simulink model "Aircraft6DSimulation"  (R2022a)
settings: Solver=FixedStepAuto  StartTime=0.0  StopTime=TF  FixedStep=dt  RelTol=1e-3
values from neighbouring files (symbols this model uses):
  a = 0    [run_model.m]
  e = 5*pi/180    (= 0.0872664625997)    [run_model.m]
  r = X(6)    [Dot_Model.m]    (also in run_model.m = out.simX.Data(:,6) * 180/pi)
  t1 = 10    [run_model.m]
  t2 = t1+2    (= 12)    [run_model.m]
  u0 = [-0.23791*pi/180 ... (first row only)    [run_model.m]
  x0 = [75 ... (first row only)    [run_model.m]
undefined symbols (not defined in the file or in its folder): Dot_Model
settings Model: Creator=Lemon  LastModifiedBy=Lemon
settings SolverCC: ZeroCrossControl=EnableAll  EnableFixedStepZeroCrossing=on

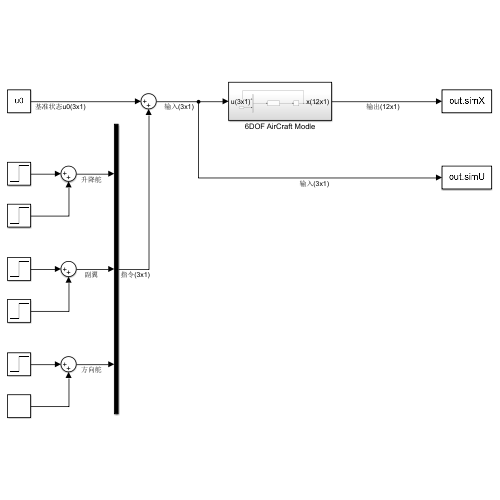
[thumbnail: Simulink's stored preview of the top-level diagram]
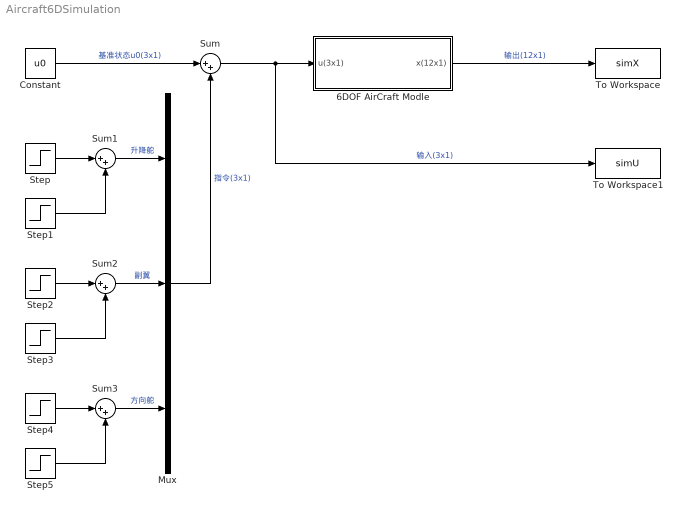
== system Aircraft6DSimulation ==
  6DOF AirCraft Modle : Subsystem
  Constant : Constant  Value=u0
  Mux : Mux  Inputs=3
  Step : Step  Time=t1  After=-e  SampleTime=0
  Step1 : Step  Time=t2  After=e  SampleTime=0
  Step2 : Step  Time=t1  After=a  SampleTime=0
  Step3 : Step  Time=t2  After=-a  SampleTime=0
  Step4 : Step  Time=t1  After=r  SampleTime=0
  Step5 : Step  Time=t2  After=-r  SampleTime=0
  Sum{,1..3} (4 alike) : Sum  Inputs=|++
  To Workspace : ToWorkspace  VariableName=simX  SaveFormat=Timeseries  SampleTime=-1
  To Workspace1 : ToWorkspace  VariableName=simU  SaveFormat=Timeseries  SampleTime=-1
  wires:
  6DOF AirCraft Modle/1(x(12x1)) -> To Workspace/1  "输出(12x1)"
  Constant/1 -> Sum/1  "基准状态u0(3x1)"
  Sum/1 -> To Workspace1/1, 6DOF AirCraft Modle/1(u(3x1))  "输入(3x1)"
  Mux/1 -> Sum/2  "指令(3x1)"
  Sum1/1 -> Mux/1  "升降舵"
  Step/1 -> Sum1/1
  Step1/1 -> Sum1/2
  Step2/1 -> Sum2/1
  Sum2/1 -> Mux/2  "副翼"
  Step3/1 -> Sum2/2
  Sum3/1 -> Mux/3  "方向舵"
  Step5/1 -> Sum3/2
  Step4/1 -> Sum3/1

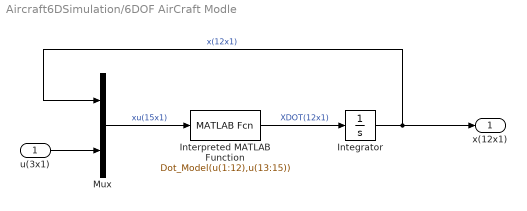
== system Aircraft6DSimulation/6DOF AirCraft Modle ==
  u(3x1) : Inport
  Integrator : Integrator  InitialCondition=x0
  Interpreted MATLAB Function : MATLABFcn  MATLABFcn=Dot_Model(u(1:12),u(13:15))
  Mux : Mux  Inputs=2
  x(12x1) : Outport
  wires:
  Mux/1 -> Interpreted MATLAB Function/1  "xu(15x1)"
  Integrator/1 -> x(12x1)/1, Mux/1  "x(12x1)"
  Interpreted MATLAB Function/1 -> Integrator/1  "XDOT(12x1)"
  u(3x1)/1 -> Mux/2
